simulink model "basic_block_soc"  (R2025a)
settings: Solver=VariableStepAuto  StartTime=0.0  StopTime=52  RelTol=1e-3
libraries: slpidlib x3, simulink x2, matrix_library x1
settings Model: Creator=manek  LastModifiedBy=manek

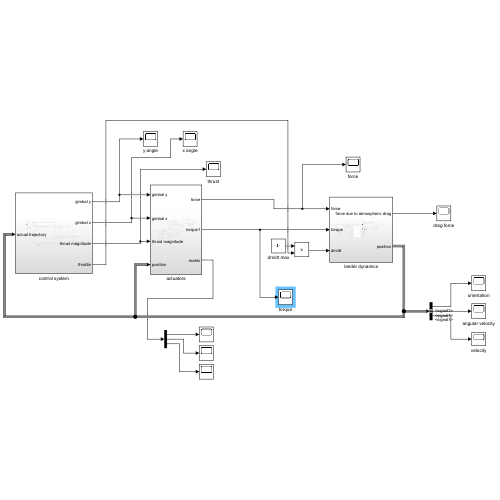
[thumbnail: Simulink's stored preview of the top-level diagram]
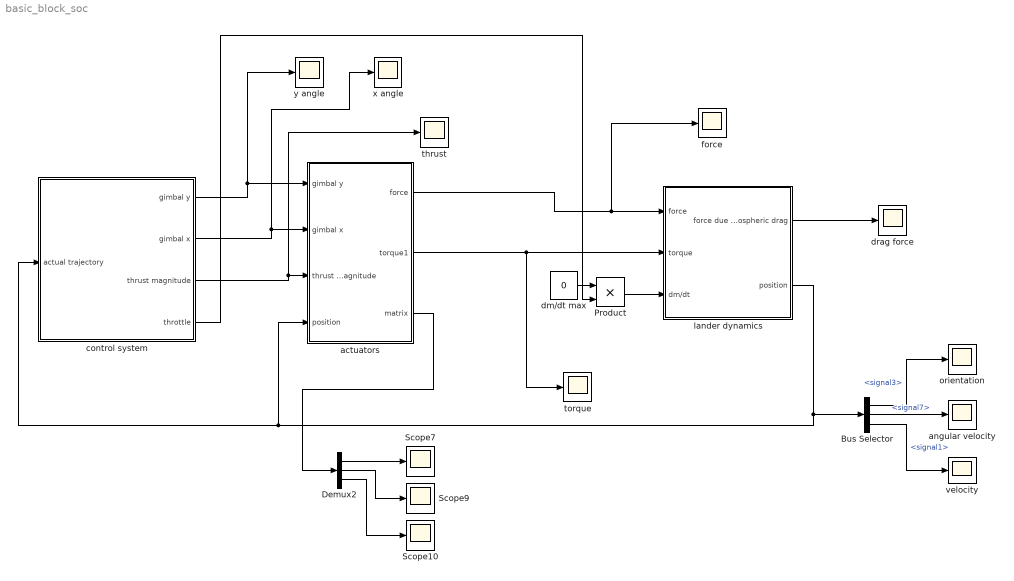
== system basic_block_soc ==
  Bus Selector : BusSelector  OutputSignals=signal3,signal7,signal1
  Demux2 : Demux  Outputs=3
  Product : Product
  Scope10 : Scope
      settings: ActiveDisplayYMinimum=-5.0082124327927513  ActiveDisplayYMaximum=4.2421969051695019  DataLoggingVariableName=ScopeData10
  Scope7 : Scope
      settings: ActiveDisplayYMinimum=-0.19463797815118633  ActiveDisplayYMaximum=0.059918312690716929  DataLoggingVariableName=ScopeData12
  Scope9 : Scope
      settings: ActiveDisplayYMinimum=-0.44705851331176949  ActiveDisplayYMaximum=0.29725794441093489  DataLoggingVariableName=ScopeData13
  actuators : Subsystem
  angular velocity : Scope
      settings: ActiveDisplayYMinimum=-0.053349523206968605  ActiveDisplayYMaximum=0.0027771393652972903  DataLoggingVariableName=ScopeData6
  control system : Subsystem
  dm/dt max : Constant  Value=0
  drag force : Scope
      settings: ActiveDisplayYMinimum=-110.31821626170756  ActiveDisplayYMaximum=678.21170399737639  DataLoggingVariableName=ScopeData4
  force : Scope
      settings: ActiveDisplayYMinimum=-6947.0885137195864  ActiveDisplayYMaximum=1420.4956935856164  DataLoggingVariableName=ScopeData14
  lander dynamics : Subsystem
  orientation : Scope
      settings: ActiveDisplayYMinimum=-0.2541390064794618  ActiveDisplayYMaximum=0.13934877849771798  DataLoggingVariableName=ScopeData3
  thrust : Scope
      settings: ActiveDisplayYMinimum=3200  ActiveDisplayYMaximum=5200  DataLoggingVariableName=ScopeData2
  torque : Scope
      settings: ActiveDisplayYMinimum=-133.21931243862662  ActiveDisplayYMaximum=56.796251258578124  DataLoggingVariableName=ScopeData11
  velocity : Scope
      settings: ActiveDisplayYMinimum=-8.0939732061337786  ActiveDisplayYMaximum=86.361865063726029  DataLoggingVariableName=ScopeData5
  x angle : Scope
      settings: ActiveDisplayYMinimum=0.0400754355875  ActiveDisplayYMaximum=0.18443606271250002
  y angle : Scope
      settings: ActiveDisplayYMinimum=-0.25597564003642159  ActiveDisplayYMaximum=0.078952091753703893
  wires:
  lander dynamics/2(position) -> control system/1(actual trajectory), actuators/4(position), Bus Selector/1
  control system/1(gimbal y) -> y angle/1, actuators/1(gimbal y)
  control system/2(gimbal x) -> x angle/1, actuators/2(gimbal x)
  control system/3(thrust magnitude) -> thrust/1, actuators/3(thrust magnitude)
  Product/1 -> lander dynamics/3(dm/dt)
  dm/dt max/1 -> Product/1
  control system/4(throttle) -> Product/2
  actuators/2(torque1) -> lander dynamics/2(torque), torque/1
  actuators/1(force) -> force/1, lander dynamics/1(force)
  Bus Selector/1 -> orientation/1  "<signal3>"
  Bus Selector/2 -> angular velocity/1  "<signal7>"
  Demux2/1 -> Scope7/1
  Demux2/2 -> Scope9/1
  Demux2/3 -> Scope10/1
  actuators/3(matrix) -> Demux2/1
  Bus Selector/3 -> velocity/1  "<signal1>"
  lander dynamics/1(force due to atmospheric drag) -> drag force/1

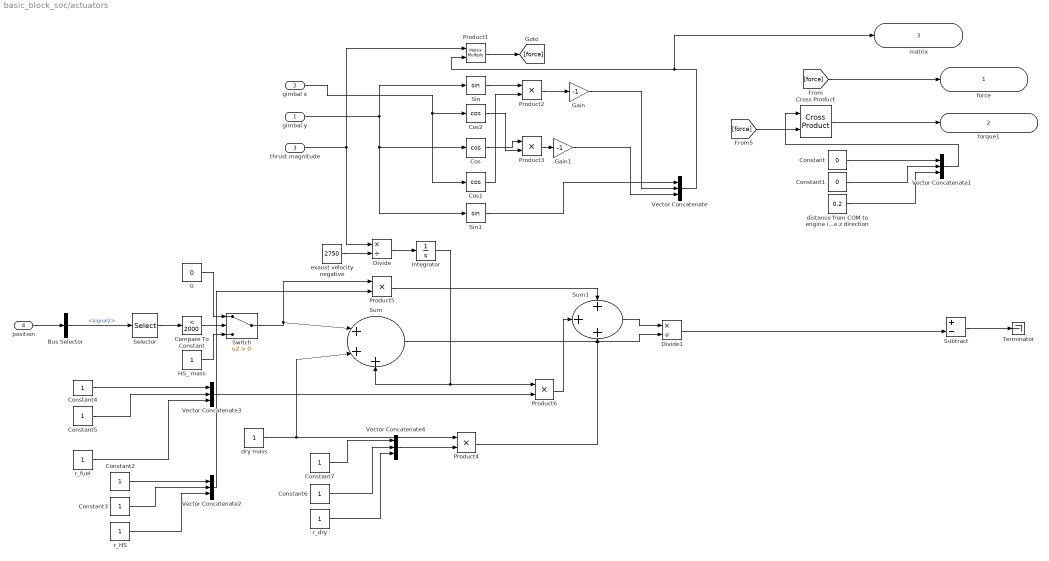
== system basic_block_soc/actuators ==
  gimbal y : Inport
  gimbal x : Inport  Port=2
  thrust magnitude : Inport  Port=3
  position : Inport  Port=4
  0 : Constant  Value=0
  Bus Selector : BusSelector  OutputSignals=signal2
  Compare To Constant : simulink/Logic and Bit Operations/Compare To Constant  relop=<  const=2000  OutDataTypeStr=boolean
  Constant : Constant  Value=0
  Constant1 : Constant  Value=0
  Constant{2..7} (6 alike) : Constant
  Cos : Trigonometry  Operator=cos
  Cos1 : Trigonometry  Operator=cos
  Cos2 : Trigonometry  Operator=cos
  Cross Product : matrix_library/Cross Product
  Divide : Product  Inputs=*/
  Divide1 : Product  Inputs=*/
  Gain : Gain  Gain=-1
  Gain1 : Gain  Gain=-1
  HS_ mass : Constant
  Integrator : Integrator  InitialCondition=50
  Product1 : Product  Multiplication=Matrix(*)
  Product{2..6} (5 alike) : Product
  Selector : Selector  InputPortWidth=3  IndexOptions=Index vector (dialog)  Indices=[3]  OutputSizes=1
  Sin : Trigonometry
  Sin1 : Trigonometry
  Subtract : Sum  Inputs=+-
  Sum : Sum  Inputs=|+++
  Sum1 : Sum  Inputs=+++
  Switch : Switch  Criteria=u2 > Threshold  SaturateOnIntegerOverflow=off  InputSameDT=off
  Terminator : Terminator
  Vector Concatenate{,1..4} (5 alike) : Concatenate  NumInputs=3
  distance from COM to engine in the negative z direction : Constant  Value=0.2
  dry mass : Constant
  exaust velocity negative : Constant  Value=2750
  r_HS : Constant
  r_dry : Constant
  r_fuel : Constant
  force : Outport  VectorParamsAs1DForOutWhenUnconnected=off
  torque1 : Outport  Port=2  VectorParamsAs1DForOutWhenUnconnected=off
  matrix : Outport  Port=3  VectorParamsAs1DForOutWhenUnconnected=off
  wires:
  Integrator/1 -> Sum/3, Product6/1
  r_fuel/1 -> Vector Concatenate3/3
  exaust velocity negative/1 -> Divide/2
  Vector Concatenate2/1 -> Product5/2
  Gain/1 -> Vector Concatenate/2
  Gain1/1 -> Vector Concatenate/3
  r_dry/1 -> Vector Concatenate4/3
  Constant2/1 -> Vector Concatenate2/1
  r_HS/1 -> Vector Concatenate2/3
  Sin/1 -> Product2/1
  Cos1/1 -> Product2/2
  gimbal x/1 -> Cos1/1, Cos2/1
  Product2/1 -> Gain/1
  Compare To Constant/1 -> Switch/2
  distance from COM to engine in the negative z direction/1 -> Vector Concatenate1/3
  [force] -> Cross Product/2
  Divide/1 -> Integrator/1
  0/1 -> Switch/1
  Sum1/1 -> Divide1/1
  Cos/1 -> Product3/1
  Sum/1 -> Divide1/2
  Product6/1 -> Sum1/2
  Product3/1 -> Gain1/1
  Cross Product/1 -> torque1/1
  Constant7/1 -> Vector Concatenate4/1
  Sin1/1 -> Vector Concatenate/1
  Vector Concatenate4/1 -> Product4/2
  Product1/1 -> [force]
  HS_ mass/1 -> Switch/3
  Constant3/1 -> Vector Concatenate2/2
  Cos2/1 -> Product3/2
  Constant1/1 -> Vector Concatenate1/2
  Vector Concatenate/1 -> matrix/1, Product1/2
  Vector Concatenate3/1 -> Product6/2
  Selector/1 -> Compare To Constant/1
  Constant4/1 -> Vector Concatenate3/1
  Product5/1 -> Sum1/1
  thrust magnitude/1 -> Product1/1, Divide/1
  Switch/1 -> Sum/1, Product5/1
  [force] -> force/1
  dry mass/1 -> Product4/1, Sum/2
  Constant5/1 -> Vector Concatenate3/2
  Constant6/1 -> Vector Concatenate4/2
  Constant/1 -> Vector Concatenate1/1
  Divide1/1 -> Subtract/2
  Product4/1 -> Sum1/3
  gimbal y/1 -> Sin/1, Sin1/1, Cos/1
  position/1 -> Bus Selector/1
  Bus Selector/1 -> Selector/1  "<signal2>"
  Vector Concatenate1/1 -> Cross Product/1
  Subtract/1 -> Terminator/1

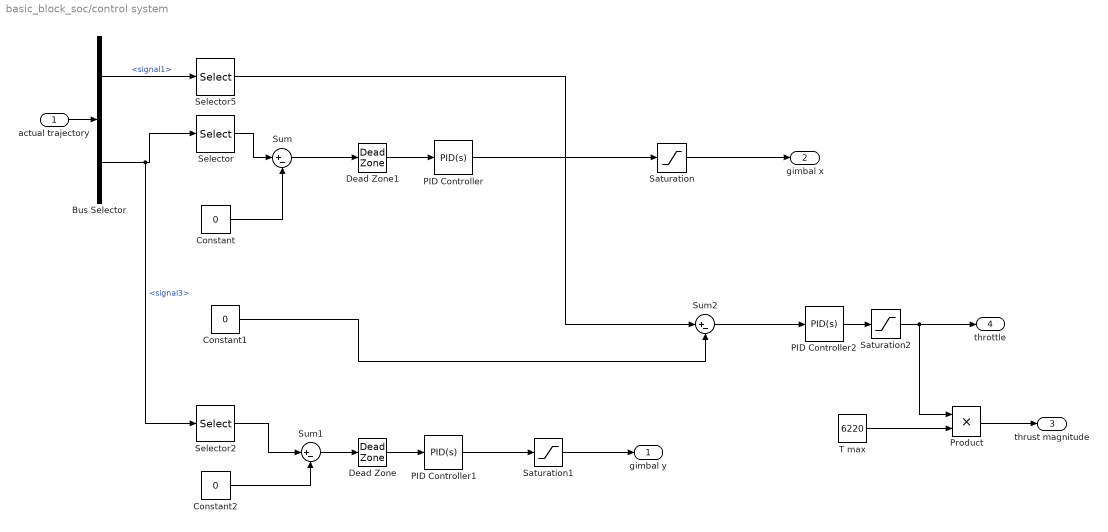
== system basic_block_soc/control system ==
  actual trajectory : Inport
  Bus Selector : BusSelector  OutputSignals=signal1,signal3
  Constant : Constant  Value=0
  Constant1 : Constant  Value=0
  Constant2 : Constant  Value=0
  Dead Zone : DeadZone  LowerValue=-0.0087  UpperValue=0.0087
  Dead Zone1 : DeadZone  LowerValue=-0.0087  UpperValue=0.0087
  PID Controller : slpidlib/PID Controller  Controller=PID  Form=Parallel  TimeDomain=Continuous-time  UseExternalTs=off  SampleTime=-1  IntegratorMethod=Forward Euler  FilterMethod=Forward Euler  ControllerParametersSource=internal  P=-1.633  I=-6.978  UseKiTs=off  D=0.02774  UseExternalDerivativeSource=off  N=8.083  UseFilter=on  TunerSelectOption=Transfer Function Based (PID Tuner App)  InitialConditionSource=internal  InitialConditionForIntegrator=0  InitialConditionForFilter=0  DifferentiatorICPrevScaledInput=0  ExternalReset=none  TrackingMode=off  Kt=1  LimitOutput=off  SatLimitsSource=internal  UpperSaturationLimit=inf  LowerSaturationLimit=-inf  LinearizeAsGain=on  AntiWindupMode=none  Kb=1  LimitIntegrator=off  UpperIntegratorSaturationLimit=inf  LowerIntegratorSaturationLimit=-inf  POutMin=[]  POutMax=[]  IOutMin=[]  IOutMax=[]  DOutMin=[]  DOutMax=[]  NOutMin=[]  NOutMax=[]  SumOutMin=[]  SumOutMax=[]  SaturationOutMin=[]  SaturationOutMax=[]  PParamMin=[]  PParamMax=[]  IParamMin=[]  IParamMax=[]  DParamMin=[]  DParamMax=[]  NParamMin=[]  NParamMax=[]  KbParamMin=[]  KbParamMax=[]  KtParamMin=[]  KtParamMax=[]  KbOutMin=[]  KbOutMax=[]  KtOutMin=[]  KtOutMax=[]  IntegratorOutMin=[]  IntegratorOutMax=[]  FilterOutMin=[]  FilterOutMax=[]  SumI1OutMin=[]  SumI1OutMax=[]  SumI2OutMin=[]  SumI2OutMax=[]  SumI3OutMin=[]  SumI3OutMax=[]  SumI4OutMin=[]  SumI4OutMax=[]  SumDOutMin=[]  SumDOutMax=[]  DifferentiatorOutMin=[]  DifferentiatorOutMax=[]  FilterDiffOutCoefMin=[]  FilterDiffOutCoefMax=[]  ReciprocalOutMin=[]  ReciprocalOutMax=[]  SumDenOutMin=[]  SumDenOutMax=[]  SumNumOutMin=[]  SumNumOutMax=[]  DivideOutMin=[]  DivideOutMax=[]  UdiffTsProdOutMin=[]  UdiffTsProdOutMax=[]  NTsProdOutMin=[]  NTsProdOutMax=[]  UintegralTsProdOutMin=[]  UintegralTsProdOutMax=[]  UngainTsProdOutMin=[]  UngainTsProdOutMax=[]  ClampingZeroOutDataTypeStr=Inherit: Inherit via back propagation  ClampingZeroOutMin=[]  ClampingZeroOutMax=[]  FilterDenConstantOutDataTypeStr=Inherit: Inherit via back propagation  FilterDenConstantOutMin=[]  FilterDenConstantOutMax=[]  PCopyOutDataTypeStr=Inherit: Inherit via back propagation  PCopyOutMin=[]  PCopyOutMax=[]  NCopyOutDataTypeStr=Inherit: Inherit via back propagation  NCopyOutMin=[]  NCopyOutMax=[]  IntegratorContinuousStateAttributes=''  IntegratorStateMustResolveToSignalObject=off  IntegratorRTWStateStorageClass=Auto  FilterContinuousStateAttributes=''  FilterStateMustResolveToSignalObject=off  FilterRTWStateStorageClass=Auto  ParallelPVariant=InternalParameters  IdealPVariant=Disabled  IVariant=InternalParameters  DVariant=InternalParameters  IntegratorVariant=Continuous  SatVariant=Disabled  AWVariant=Passthrough  PCopyVariant=Disabled  TRVariant=Disabled  FdbkBlocksVariant=Forward  IdealPFdbkVariant=Disabled  SatFdbkVariant=Disabled  DerivativeFilterVariant=ContFilter  NVariant=InternalParameters  NCopyVariant=Disabled  FilterICVariant=InternalICsFilter  IntegratorICVariant=InternalICs  ExternalResetVariant=Disabled  TRSumVariant=Passthrough  SumFdbkVariant=Disabled  SumVariant=Sum_PID  TsampFilterVariant=InternalTs  TsampNgainVariant=Passthrough  TsampIntegralVariant=Disabled_SignalSpec  ExternalSaturationOutDataTypeStr=Inherit: Same as second input  DerivativeSourceVariant=ErrorSignal  PreIntVariant=InternalPreInt
  PID Controller1 : slpidlib/PID Controller  Controller=PID  Form=Parallel  TimeDomain=Continuous-time  UseExternalTs=off  SampleTime=-1  IntegratorMethod=Forward Euler  FilterMethod=Forward Euler  ControllerParametersSource=internal  P=-0.787154990138742  I=-0.0740260738755154  UseKiTs=off  D=-2.05339357900365  UseExternalDerivativeSource=off  N=10.392326076349  UseFilter=on  TunerSelectOption=Transfer Function Based (PID Tuner App)  InitialConditionSource=internal  InitialConditionForIntegrator=0  InitialConditionForFilter=0  DifferentiatorICPrevScaledInput=0  ExternalReset=none  TrackingMode=off  Kt=1  LimitOutput=off  SatLimitsSource=internal  UpperSaturationLimit=inf  LowerSaturationLimit=-inf  LinearizeAsGain=on  AntiWindupMode=none  Kb=1  LimitIntegrator=off  UpperIntegratorSaturationLimit=inf  LowerIntegratorSaturationLimit=-inf  POutMin=[]  POutMax=[]  IOutMin=[]  IOutMax=[]  DOutMin=[]  DOutMax=[]  NOutMin=[]  NOutMax=[]  SumOutMin=[]  SumOutMax=[]  SaturationOutMin=[]  SaturationOutMax=[]  PParamMin=[]  PParamMax=[]  IParamMin=[]  IParamMax=[]  DParamMin=[]  DParamMax=[]  NParamMin=[]  NParamMax=[]  KbParamMin=[]  KbParamMax=[]  KtParamMin=[]  KtParamMax=[]  KbOutMin=[]  KbOutMax=[]  KtOutMin=[]  KtOutMax=[]  IntegratorOutMin=[]  IntegratorOutMax=[]  FilterOutMin=[]  FilterOutMax=[]  SumI1OutMin=[]  SumI1OutMax=[]  SumI2OutMin=[]  SumI2OutMax=[]  SumI3OutMin=[]  SumI3OutMax=[]  SumI4OutMin=[]  SumI4OutMax=[]  SumDOutMin=[]  SumDOutMax=[]  DifferentiatorOutMin=[]  DifferentiatorOutMax=[]  FilterDiffOutCoefMin=[]  FilterDiffOutCoefMax=[]  ReciprocalOutMin=[]  ReciprocalOutMax=[]  SumDenOutMin=[]  SumDenOutMax=[]  SumNumOutMin=[]  SumNumOutMax=[]  DivideOutMin=[]  DivideOutMax=[]  UdiffTsProdOutMin=[]  UdiffTsProdOutMax=[]  NTsProdOutMin=[]  NTsProdOutMax=[]  UintegralTsProdOutMin=[]  UintegralTsProdOutMax=[]  UngainTsProdOutMin=[]  UngainTsProdOutMax=[]  ClampingZeroOutDataTypeStr=Inherit: Inherit via back propagation  ClampingZeroOutMin=[]  ClampingZeroOutMax=[]  FilterDenConstantOutDataTypeStr=Inherit: Inherit via back propagation  FilterDenConstantOutMin=[]  FilterDenConstantOutMax=[]  PCopyOutDataTypeStr=Inherit: Inherit via back propagation  PCopyOutMin=[]  PCopyOutMax=[]  NCopyOutDataTypeStr=Inherit: Inherit via back propagation  NCopyOutMin=[]  NCopyOutMax=[]  IntegratorContinuousStateAttributes=''  IntegratorStateMustResolveToSignalObject=off  IntegratorRTWStateStorageClass=Auto  FilterContinuousStateAttributes=''  FilterStateMustResolveToSignalObject=off  FilterRTWStateStorageClass=Auto  ParallelPVariant=InternalParameters  IdealPVariant=Disabled  IVariant=InternalParameters  DVariant=InternalParameters  IntegratorVariant=Continuous  SatVariant=Disabled  AWVariant=Passthrough  PCopyVariant=Disabled  TRVariant=Disabled  FdbkBlocksVariant=Forward  IdealPFdbkVariant=Disabled  SatFdbkVariant=Disabled  DerivativeFilterVariant=ContFilter  NVariant=InternalParameters  NCopyVariant=Disabled  FilterICVariant=InternalICsFilter  IntegratorICVariant=InternalICs  ExternalResetVariant=Disabled  TRSumVariant=Passthrough  SumFdbkVariant=Disabled  SumVariant=Sum_PID  TsampFilterVariant=InternalTs  TsampNgainVariant=Passthrough  TsampIntegralVariant=Disabled_SignalSpec  ExternalSaturationOutDataTypeStr=Inherit: Same as second input  DerivativeSourceVariant=ErrorSignal  PreIntVariant=InternalPreInt
  PID Controller2 : slpidlib/PID Controller  Controller=PID  Form=Parallel  TimeDomain=Continuous-time  UseExternalTs=off  SampleTime=-1  IntegratorMethod=Forward Euler  FilterMethod=Forward Euler  ControllerParametersSource=internal  P=0.00677902593089405  I=0.00121493023367645  UseKiTs=off  D=0  UseExternalDerivativeSource=off  N=100  UseFilter=on  TunerSelectOption=Transfer Function Based (PID Tuner App)  InitialConditionSource=internal  InitialConditionForIntegrator=0  InitialConditionForFilter=0  DifferentiatorICPrevScaledInput=0  ExternalReset=none  TrackingMode=off  Kt=1  LimitOutput=off  SatLimitsSource=internal  UpperSaturationLimit=inf  LowerSaturationLimit=-inf  LinearizeAsGain=on  AntiWindupMode=none  Kb=1  LimitIntegrator=off  UpperIntegratorSaturationLimit=inf  LowerIntegratorSaturationLimit=-inf  POutMin=[]  POutMax=[]  IOutMin=[]  IOutMax=[]  DOutMin=[]  DOutMax=[]  NOutMin=[]  NOutMax=[]  SumOutMin=[]  SumOutMax=[]  SaturationOutMin=[]  SaturationOutMax=[]  PParamMin=[]  PParamMax=[]  IParamMin=[]  IParamMax=[]  DParamMin=[]  DParamMax=[]  NParamMin=[]  NParamMax=[]  KbParamMin=[]  KbParamMax=[]  KtParamMin=[]  KtParamMax=[]  KbOutMin=[]  KbOutMax=[]  KtOutMin=[]  KtOutMax=[]  IntegratorOutMin=[]  IntegratorOutMax=[]  FilterOutMin=[]  FilterOutMax=[]  SumI1OutMin=[]  SumI1OutMax=[]  SumI2OutMin=[]  SumI2OutMax=[]  SumI3OutMin=[]  SumI3OutMax=[]  SumI4OutMin=[]  SumI4OutMax=[]  SumDOutMin=[]  SumDOutMax=[]  DifferentiatorOutMin=[]  DifferentiatorOutMax=[]  FilterDiffOutCoefMin=[]  FilterDiffOutCoefMax=[]  ReciprocalOutMin=[]  ReciprocalOutMax=[]  SumDenOutMin=[]  SumDenOutMax=[]  SumNumOutMin=[]  SumNumOutMax=[]  DivideOutMin=[]  DivideOutMax=[]  UdiffTsProdOutMin=[]  UdiffTsProdOutMax=[]  NTsProdOutMin=[]  NTsProdOutMax=[]  UintegralTsProdOutMin=[]  UintegralTsProdOutMax=[]  UngainTsProdOutMin=[]  UngainTsProdOutMax=[]  ClampingZeroOutDataTypeStr=Inherit: Inherit via back propagation  ClampingZeroOutMin=[]  ClampingZeroOutMax=[]  FilterDenConstantOutDataTypeStr=Inherit: Inherit via back propagation  FilterDenConstantOutMin=[]  FilterDenConstantOutMax=[]  PCopyOutDataTypeStr=Inherit: Inherit via back propagation  PCopyOutMin=[]  PCopyOutMax=[]  NCopyOutDataTypeStr=Inherit: Inherit via back propagation  NCopyOutMin=[]  NCopyOutMax=[]  IntegratorContinuousStateAttributes=''  IntegratorStateMustResolveToSignalObject=off  IntegratorRTWStateStorageClass=Auto  FilterContinuousStateAttributes=''  FilterStateMustResolveToSignalObject=off  FilterRTWStateStorageClass=Auto  ParallelPVariant=InternalParameters  IdealPVariant=Disabled  IVariant=InternalParameters  DVariant=InternalParameters  IntegratorVariant=Continuous  SatVariant=Disabled  AWVariant=Passthrough  PCopyVariant=Disabled  TRVariant=Disabled  FdbkBlocksVariant=Forward  IdealPFdbkVariant=Disabled  SatFdbkVariant=Disabled  DerivativeFilterVariant=ContFilter  NVariant=InternalParameters  NCopyVariant=Disabled  FilterICVariant=InternalICsFilter  IntegratorICVariant=InternalICs  ExternalResetVariant=Disabled  TRSumVariant=Passthrough  SumFdbkVariant=Disabled  SumVariant=Sum_PID  TsampFilterVariant=InternalTs  TsampNgainVariant=Passthrough  TsampIntegralVariant=Disabled_SignalSpec  ExternalSaturationOutDataTypeStr=Inherit: Same as second input  DerivativeSourceVariant=ErrorSignal  PreIntVariant=InternalPreInt
  Product : Product
  Saturation : Saturate  UpperLimit=0.17  LowerLimit=-0.17
  Saturation1 : Saturate  UpperLimit=0.17  LowerLimit=-0.17
  Saturation2 : Saturate  UpperLimit=1  LowerLimit=0
  Selector : Selector  InputPortWidth=3  IndexOptions=Index vector (dialog)  Indices=[1]  OutputSizes=1
  Selector2 : Selector  InputPortWidth=3  IndexOptions=Index vector (dialog)  Indices=[2]  OutputSizes=1
  Selector5 : Selector  InputPortWidth=3  IndexOptions=Index vector (dialog)  Indices=[3]  OutputSizes=1
  Sum : Sum  Inputs=|+-
  Sum1 : Sum  Inputs=|+-
  Sum2 : Sum  Inputs=|+-
  T max : Constant  Value=6220
  gimbal y : Outport
  gimbal x : Outport  Port=2
  thrust magnitude : Outport  Port=3
  throttle : Outport  Port=4
  wires:
  actual trajectory/1 -> Bus Selector/1
  Selector/1 -> Sum/1
  Constant/1 -> Sum/2
  Selector2/1 -> Sum1/1
  Constant2/1 -> Sum1/2
  Sum/1 -> Dead Zone1/1
  PID Controller/1 -> Saturation/1
  Sum1/1 -> Dead Zone/1
  PID Controller1/1 -> Saturation1/1
  Bus Selector/1 -> Selector5/1  "<signal1>"
  Sum2/1 -> PID Controller2/1
  PID Controller2/1 -> Saturation2/1
  T max/1 -> Product/2
  Product/1 -> thrust magnitude/1
  Saturation/1 -> gimbal x/1
  Saturation1/1 -> gimbal y/1
  Constant1/1 -> Sum2/2
  Selector5/1 -> Sum2/1
  Saturation2/1 -> Product/1, throttle/1
  Bus Selector/2 -> Selector2/1, Selector/1  "<signal3>"
  Dead Zone/1 -> PID Controller1/1
  Dead Zone1/1 -> PID Controller/1

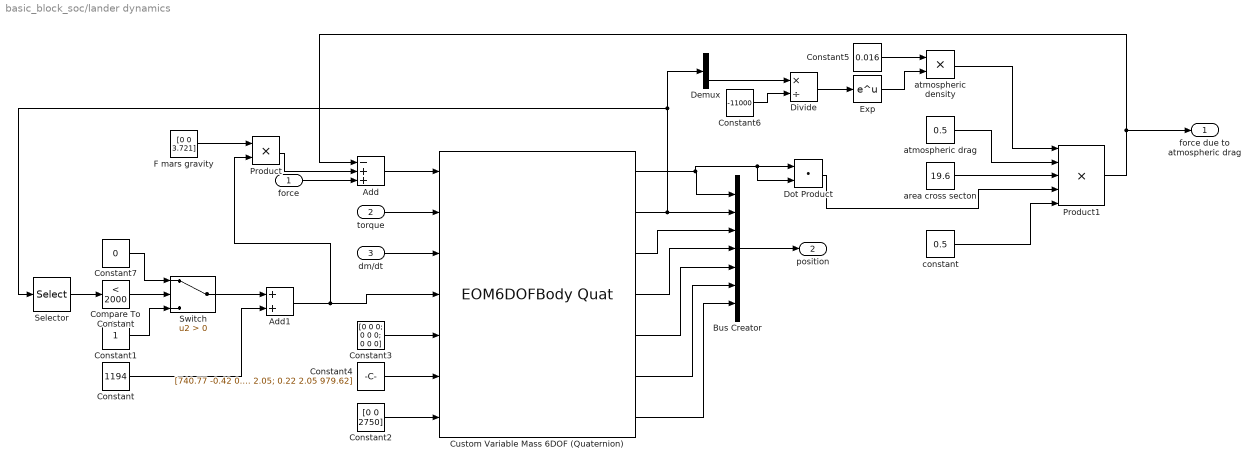
== system basic_block_soc/lander dynamics ==
  force : Inport
  torque : Inport  Port=2
  dm/dt : Inport  Port=3
  Add : Sum  Inputs=-++
  Add1 : Sum
  Bus Creator : BusCreator  Inputs=7
  Compare To Constant : simulink/Logic and Bit Operations/Compare To Constant  relop=<  const=2000  OutDataTypeStr=boolean
  Constant : Constant  Value=1194
  Constant1 : Constant
  Constant2 : Constant  Value=[0 0 2750]
  Constant3 : Constant  Value=[0 0 0; 0 0 0; 0 0 0]  OutDataTypeStr=double
  Constant4 : Constant  Value=[740.77 -0.42 0.22; -0.42 710.41 2.05; 0.22 2.05 979.62]  OutDataTypeStr=double
  Constant5 : Constant  Value=0.016
  Constant6 : Constant  Value=-11000
  Constant7 : Constant  Value=0
  Custom Variable Mass 6DOF (Quaternion) : EOM6DOFBodyQuat  mtype=Custom Variable  xme_0=[0 0 -2000]  Vm_0=[0 0 77]  eul_0=[0.05 0.1 0]  vre_flag=on
  Demux : Demux  Outputs=3
  Divide : Product  Inputs=*/
  Dot Product : DotProduct  OutDataTypeStr=Inherit: Inherit via internal rule
  Exp : Math
  F mars gravity : Constant  Value=[0 0 3.721]
  Product : Product
  Product1 : Product  Inputs=5
  Selector : Selector  InputPortWidth=3  IndexOptions=Index vector (dialog)  Indices=[3]  OutputSizes=1
  Switch : Switch  Criteria=u2 > Threshold  SaturateOnIntegerOverflow=off  InputSameDT=off
  area cross secton : Constant  Value=19.6
  atmospheric density : Product
  atmospheric drag : Constant  Value=0.5
  constant : Constant  Value=0.5
  force due to atmospheric drag : Outport
  position : Outport  Port=2
  wires:
  Constant2/1 -> Custom Variable Mass 6DOF (Quaternion)/7
  Constant3/1 -> Custom Variable Mass 6DOF (Quaternion)/5
  dm/dt/1 -> Custom Variable Mass 6DOF (Quaternion)/3
  Bus Creator/1 -> position/1
  Custom Variable Mass 6DOF (Quaternion)/1 -> Dot Product/2, Dot Product/1, Bus Creator/1
  Custom Variable Mass 6DOF (Quaternion)/2 -> Bus Creator/2, Demux/1, Selector/1
  Custom Variable Mass 6DOF (Quaternion)/3 -> Bus Creator/3
  Custom Variable Mass 6DOF (Quaternion)/4 -> Bus Creator/4
  Custom Variable Mass 6DOF (Quaternion)/5 -> Bus Creator/5
  Custom Variable Mass 6DOF (Quaternion)/6 -> Bus Creator/6
  Custom Variable Mass 6DOF (Quaternion)/7 -> Bus Creator/7
  Constant4/1 -> Custom Variable Mass 6DOF (Quaternion)/6
  F mars gravity/1 -> Product/1
  torque/1 -> Custom Variable Mass 6DOF (Quaternion)/2
  Product/1 -> Add/2
  force/1 -> Add/3
  Add/1 -> Custom Variable Mass 6DOF (Quaternion)/1
  Constant5/1 -> atmospheric density/1
  Demux/3 -> Divide/1
  Constant6/1 -> Divide/2
  Divide/1 -> Exp/1
  Exp/1 -> atmospheric density/2
  Constant1/1 -> Switch/3
  Constant7/1 -> Switch/1
  Compare To Constant/1 -> Switch/2
  Selector/1 -> Compare To Constant/1
  atmospheric density/1 -> Product1/1
  atmospheric drag/1 -> Product1/2
  area cross secton/1 -> Product1/3
  constant/1 -> Product1/5
  Dot Product/1 -> Product1/4
  Product1/1 -> Add/1, force due to atmospheric drag/1
  Switch/1 -> Add1/1
  Constant/1 -> Add1/2
  Add1/1 -> Product/2, Custom Variable Mass 6DOF (Quaternion)/4
